simulink model "test_01_3d_veh_piby567_2018"  (R2018a)
settings: Solver=FixedStepAuto  StartTime=0.0  StopTime=50  FixedStep=0.1  RelTol=1e-3
values from neighbouring files (symbols this model uses):
  boundary = 0.1    [piby5tunnel.m]
  d_star = 0.6    [piby5tunnel.m]
  delta_arrow = 0.0295    [piby5tunnel.m]
  dtr = 7.3    [piby5tunnel.m]
  mu = 0.1    [piby5tunnel.m]
  N_n_p = zeros(slice,3)    [piby5tunnel.m]
  N_nfinal = zeros(slice-1,3*sides)    [piby5tunnel.m]
  P_c_final = zeros(slice-1,3*sides)    [piby5tunnel.m]
  sides = 8    [piby5tunnel.m]
  sigma = 0.005    [piby5tunnel.m]
  sum_ovf = zeros(slice,3)    [piby5tunnel.m]
  ubar = 1.5    [piby5tunnel.m]
  Ud = 1.485    [piby5tunnel.m]
  us = 1    [piby5tunnel.m]
  Vd = 1    [piby5tunnel.m]
  vehicle_velocity = 1    [piby5tunnel.m]
  x_0 = 30    [piby5tunnel.m]
  y_0 = 0    [piby5tunnel.m]
  z_0 = 0    [piby5tunnel.m]
libraries: vrlib x1, simulink x1
settings Model: Creator=satis  LastModifiedBy=Rasmus Visgaard

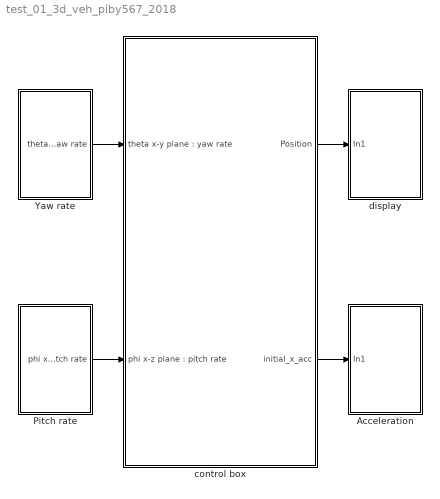
== system test_01_3d_veh_piby567_2018 ==
  "Acceleration " : Subsystem
  Pitch rate : Subsystem
  Yaw rate : Subsystem
  control box : Subsystem
  display : Subsystem
  wires:
  control box/1(Position) -> display/1(In1)
  Yaw rate/1("theta x-y plane : yaw rate") -> control box/1("theta x-y plane : yaw rate")
  Pitch rate/1("phi x-z plane : pitch rate") -> control box/2("phi x-z plane : pitch rate")
  control box/2(initial_x_acc) -> "Acceleration "/1(In1)

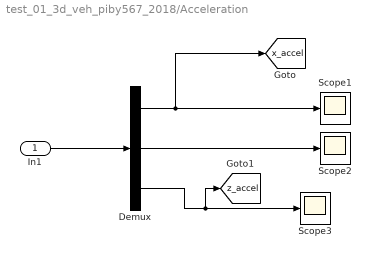
== system test_01_3d_veh_piby567_2018/Acceleration  ==
  In1 : Inport
  Demux : Demux  Outputs=3
  Scope1 : Scope
  Scope2 : Scope
  Scope3 : Scope
  tag scope: x_accel=global, z_accel=global
  wires:
  Demux/2 -> Scope2/1
  Demux/1 -> [x_accel], Scope1/1
  Demux/3 -> [z_accel], Scope3/1
  In1/1 -> Demux/1

== system test_01_3d_veh_piby567_2018/Pitch rate ==
  Constant4 : Constant  Value=0
  Step1 : Step  Time=0.1  SampleTime=0
  Switch1 : Switch  Criteria=u2 > Threshold
  "phi x-z plane : pitch rate" : Outport  VectorParamsAs1DForOutWhenUnconnected=off
  wires:
  Step1/1 -> Switch1/2
  Constant4/1 -> Switch1/3  "theta x-z plane : pitch rate"
  Switch1/1 -> "phi x-z plane : pitch rate"/1  "phi x-z plane : pitch rate"
  [z_accel] -> Switch1/1

== system test_01_3d_veh_piby567_2018/Yaw rate ==
  Constant2 : Constant  Value=0
  Step : Step  Time=0.1  SampleTime=0
  Switch : Switch  Criteria=u2 > Threshold
  "theta x-y plane : yaw rate" : Outport  VectorParamsAs1DForOutWhenUnconnected=off
  wires:
  Switch/1 -> "theta x-y plane : yaw rate"/1  "theta x-y plane : yaw rate"
  [x_accel] -> Switch/1
  Constant2/1 -> Switch/3  "theta x-y plane : yaw rate"
  Step/1 -> Switch/2

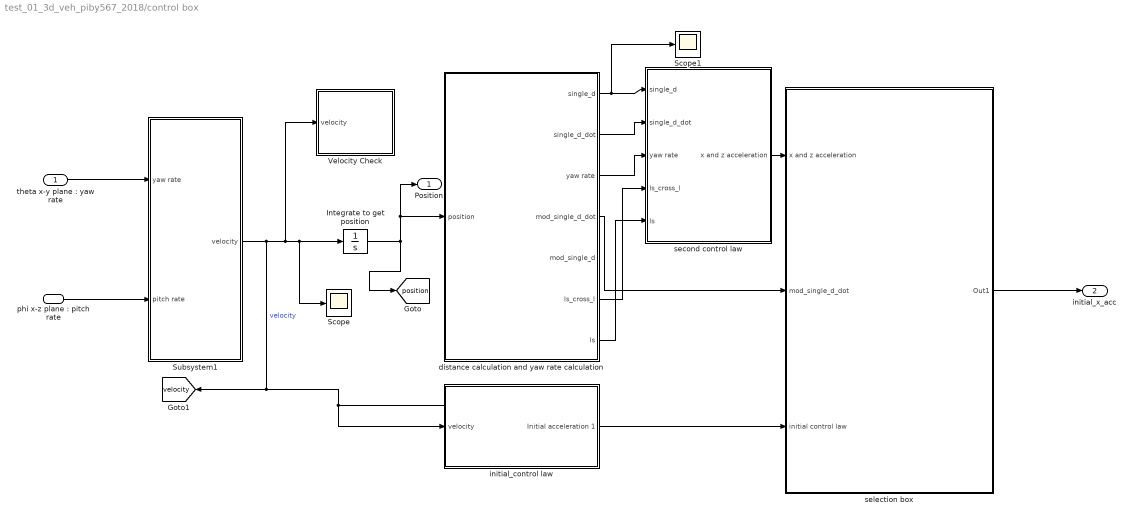
== system test_01_3d_veh_piby567_2018/control box ==
  "theta x-y plane : yaw rate" : Inport
  "phi x-z plane : pitch rate" : Inport  Port=2
  Integrate to get position : Integrator  InitialCondition=[x_0 z_0 y_0]
  Scope : Scope
  Scope1 : Scope
  Subsystem1 : Subsystem
  "Velocity Check " : Subsystem
  "distance calculation and yaw rate calculation " : Subsystem
  initial_control law : Subsystem
  second control law : Subsystem
  "selection box " : Subsystem
  Position : Outport  VectorParamsAs1DForOutWhenUnconnected=off
  initial_x_acc : Outport  Port=2  VectorParamsAs1DForOutWhenUnconnected=off
  tag scope: position=global, velocity=global
  wires:
  Subsystem1/1(velocity) -> initial_control law/1(velocity), [velocity], Scope/1, Integrate to get position/1, "Velocity Check "/1(velocity)  "velocity"
  "theta x-y plane : yaw rate"/1 -> Subsystem1/1("yaw rate ")
  "phi x-z plane : pitch rate"/1 -> Subsystem1/2(pitch rate)
  Integrate to get position/1 -> [position], Position/1, "distance calculation and yaw rate calculation "/1(position)
  "selection box "/1(Out1) -> initial_x_acc/1
  second control law/1(x and z acceleration) -> "selection box "/1(x and z acceleration)
  "distance calculation and yaw rate calculation "/1(single_d) -> Scope1/1, second control law/1(single_d)
  "distance calculation and yaw rate calculation "/2(single_d_dot) -> second control law/2(single_d_dot)
  "distance calculation and yaw rate calculation "/4(mod_single_d_dot) -> "selection box "/2(mod_single_d_dot)
  "distance calculation and yaw rate calculation "/3(yaw rate) -> second control law/3(yaw rate)
  "distance calculation and yaw rate calculation "/6(ls_cross_l) -> second control law/4(ls_cross_l)
  "distance calculation and yaw rate calculation "/7(ls) -> second control law/5(ls)
  initial_control law/1(Initial acceleration 1) -> "selection box "/3(initial control law)

== system test_01_3d_veh_piby567_2018/display ==
  In1 : Inport
  Demux : Demux  Outputs=3
  Scope10 : Scope
  Scope11 : Scope
  Scope12 : Scope
  wires:
  Demux/1 -> Scope10/1
  Demux/2 -> Scope11/1
  Demux/3 -> Scope12/1
  In1/1 -> Demux/1

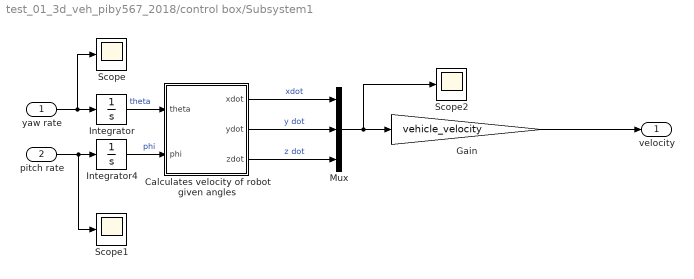
== system test_01_3d_veh_piby567_2018/control box/Subsystem1 ==
  "yaw rate " : Inport
  pitch rate : Inport  Port=2
  Calculates velocity of robot given angles : MATLAB Function  TreatAsAtomicUnit=on
  Gain : Gain  Gain=vehicle_velocity
  Integrator : Integrator
  Integrator4 : Integrator
  Mux : Mux  Inputs=3
  Scope : Scope
  Scope1 : Scope
  Scope2 : Scope
  velocity : Outport  VectorParamsAs1DForOutWhenUnconnected=off
  wires:
  Integrator4/1 -> Calculates velocity of robot given angles/2(phi)  "phi"
  Calculates velocity of robot given angles/1(xdot) -> Mux/1  "xdot"
  Integrator/1 -> Calculates velocity of robot given angles/1(theta)  "theta"
  Calculates velocity of robot given angles/2(ydot) -> Mux/2  "y dot"
  pitch rate/1 -> Scope1/1, Integrator4/1
  "yaw rate "/1 -> Scope/1, Integrator/1
  Calculates velocity of robot given angles/3(zdot) -> Mux/3  "z dot"
  Gain/1 -> velocity/1
  Mux/1 -> Scope2/1, Gain/1

== system test_01_3d_veh_piby567_2018/control box/Velocity Check  ==
  velocity : Inport
  Scope : Scope
  norm of velocity : Subsystem
  wires:
  norm of velocity/1(Out1) -> Scope/1
  velocity/1 -> norm of velocity/1(In1)

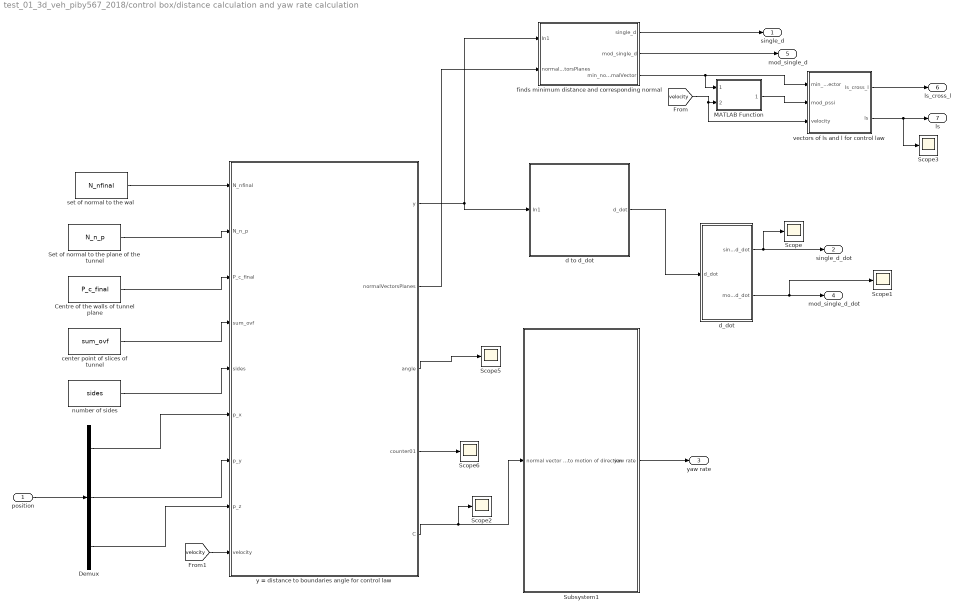
== system test_01_3d_veh_piby567_2018/control box/distance calculation and yaw rate calculation  ==
  position : Inport
  Centre of the walls of tunnel plane : Constant  Value=P_c_final  VectorParams1D=off
  Demux : Demux  Outputs=3
  MATLAB Function : MATLAB Function  TreatAsAtomicUnit=on
  Scope{,1..3,5..6} (6 alike) : Scope
  Set of normal to the plane of the tunnel : Constant  Value=N_n_p  VectorParams1D=off
  Subsystem1 : Subsystem
  center point of slices of tunnel : Constant  Value=sum_ovf  VectorParams1D=off
  d to d_dot : Subsystem
  d_dot : Subsystem
  finds minimum distance and corresponding normal : Subsystem
  number of sides : Constant  Value=sides
  set of normal to the wal : Constant  Value=N_nfinal  VectorParams1D=off
  vectors of ls and l for control law : MATLAB Function  TreatAsAtomicUnit=on
  "y = distance to boundaries angle for control law " : MATLAB Function  TreatAsAtomicUnit=on
  single_d : Outport  VectorParamsAs1DForOutWhenUnconnected=off
  single_d_dot : Outport  Port=2  VectorParamsAs1DForOutWhenUnconnected=off
  yaw rate : Outport  Port=3  VectorParamsAs1DForOutWhenUnconnected=off
  mod_single_d_dot : Outport  Port=4  VectorParamsAs1DForOutWhenUnconnected=off
  mod_single_d : Outport  Port=5  VectorParamsAs1DForOutWhenUnconnected=off
  ls_cross_l : Outport  Port=6
  ls : Outport  Port=7
  wires:
  set of normal to the wal/1 -> "y = distance to boundaries angle for control law "/1(N_nfinal)
  Centre of the walls of tunnel plane/1 -> "y = distance to boundaries angle for control law "/3(P_c_final)
  Set of normal to the plane of the tunnel/1 -> "y = distance to boundaries angle for control law "/2(N_n_p)
  center point of slices of tunnel/1 -> "y = distance to boundaries angle for control law "/4(sum_ovf)
  number of sides/1 -> "y = distance to boundaries angle for control law "/5(sides)
  position/1 -> Demux/1
  "y = distance to boundaries angle for control law "/1(y) -> d to d_dot/1(In1), finds minimum distance and corresponding normal/1(In1)
  Demux/1 -> "y = distance to boundaries angle for control law "/6(p_x)
  Demux/2 -> "y = distance to boundaries angle for control law "/7(p_y)
  Demux/3 -> "y = distance to boundaries angle for control law "/8(p_z)
  d to d_dot/1(d_dot) -> d_dot/1(d_dot)
  "y = distance to boundaries angle for control law "/3(angle) -> Scope5/1
  "y = distance to boundaries angle for control law "/4(counter01) -> Scope6/1
  "y = distance to boundaries angle for control law "/5(C) -> Scope2/1, Subsystem1/1(normal vector to motion of direction)
  Subsystem1/1(yaw rate) -> yaw rate/1
  finds minimum distance and corresponding normal/1(single_d) -> single_d/1
  finds minimum distance and corresponding normal/2(mod_single_d) -> mod_single_d/1
  d_dot/1(single_d_dot) -> Scope/1, single_d_dot/1
  d_dot/2(mod_single_d_dot) -> Scope1/1, mod_single_d_dot/1
  "y = distance to boundaries angle for control law "/2(normalVectorsPlanes) -> finds minimum distance and corresponding normal/2(normalVectorsPlanes)
  finds minimum distance and corresponding normal/3(min_normalVector) -> vectors of ls and l for control law/1(min_normalVector), MATLAB Function/1(min_normalVector)
  [velocity] -> MATLAB Function/2(velocity), vectors of ls and l for control law/3(velocity)
  MATLAB Function/1(mod_pssi) -> vectors of ls and l for control law/2(mod_pssi)
  vectors of ls and l for control law/1(ls_cross_l) -> ls_cross_l/1
  vectors of ls and l for control law/2(ls) -> Scope3/1, ls/1
  [velocity] -> "y = distance to boundaries angle for control law "/9(velocity)

== system test_01_3d_veh_piby567_2018/control box/initial_control law ==
  velocity : Inport
  Constant2 : Constant  Value=initial_normal_vector'
  Cross Product : vrlib/Utilities/Cross Product
      settings: SourceProductName=Simulink
  Gain : Gain  Gain=ubar
  Initial acceleration 1 : Outport  VectorParamsAs1DForOutWhenUnconnected=off
  wires:
  Cross Product/1 -> Gain/1
  velocity/1 -> Cross Product/1
  Constant2/1 -> Cross Product/2
  Gain/1 -> Initial acceleration 1/1

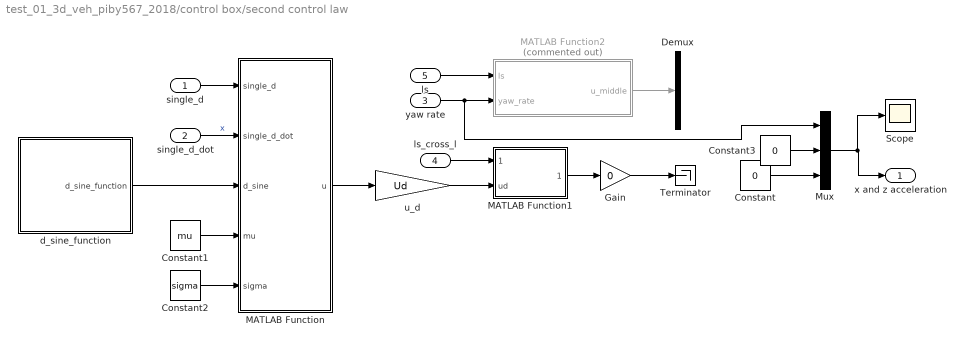
== system test_01_3d_veh_piby567_2018/control box/second control law ==
  single_d : Inport
  single_d_dot : Inport  Port=2
  yaw rate : Inport  Port=3
  ls_cross_l : Inport  Port=4
  ls : Inport  Port=5
  Constant : Constant  Value=0
  Constant1 : Constant  Value=mu
  Constant2 : Constant  Value=sigma
  Constant3 : Constant  Value=0
  Demux : Demux  Outputs=3
  Gain : Gain  Gain=0
  MATLAB Function : MATLAB Function  TreatAsAtomicUnit=on
  MATLAB Function1 : MATLAB Function  TreatAsAtomicUnit=on
  MATLAB Function2 : MATLAB Function  Commented=on  TreatAsAtomicUnit=on
  Mux : Mux  Inputs=3
  Scope : Scope
  Terminator : Terminator
  d_sine_function : Subsystem
  u_d : Gain  Gain=Ud
  x and z acceleration : Outport  VectorParamsAs1DForOutWhenUnconnected=off
  wires:
  single_d/1 -> MATLAB Function/1(single_d)
  Constant1/1 -> MATLAB Function/4(mu)
  Constant2/1 -> MATLAB Function/5(sigma)
  MATLAB Function/1(u) -> u_d/1
  d_sine_function/1(d_sine_function) -> MATLAB Function/3(d_sine)
  single_d_dot/1 -> MATLAB Function/2(single_d_dot)  "x"
  u_d/1 -> MATLAB Function1/2(ud)
  ls_cross_l/1 -> MATLAB Function1/1(ls_cross_l)
  ls/1 -> MATLAB Function2/1(ls)
  yaw rate/1 -> Mux/1, MATLAB Function2/2(yaw_rate)
  MATLAB Function2/1(u_middle) -> Demux/1
  MATLAB Function1/1(u_boundary) -> Gain/1
  Gain/1 -> Terminator/1
  Constant/1 -> Mux/3
  Constant3/1 -> Mux/2
  Mux/1 -> Scope/1, x and z acceleration/1

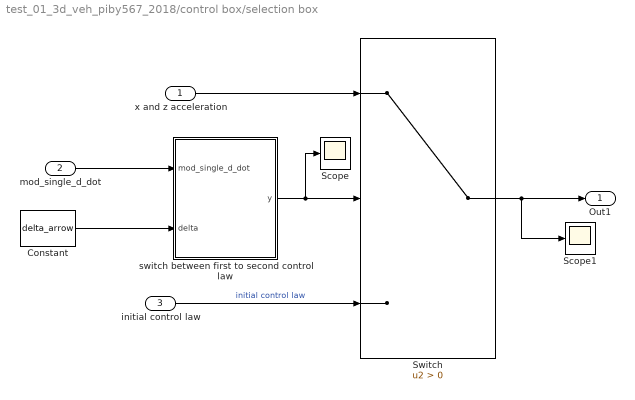
== system test_01_3d_veh_piby567_2018/control box/selection box  ==
  x and z acceleration : Inport
  mod_single_d_dot : Inport  Port=2
  initial control law : Inport  Port=3
  Constant : Constant  Value=delta_arrow
  Scope : Scope
  Scope1 : Scope
  Switch : Switch  Criteria=u2 > Threshold
  switch between first to second control law : MATLAB Function  TreatAsAtomicUnit=on
  Out1 : Outport  VectorParamsAs1DForOutWhenUnconnected=off
  wires:
  initial control law/1 -> Switch/3  "initial control law"
  x and z acceleration/1 -> Switch/1
  Constant/1 -> switch between first to second control law/2(delta)
  mod_single_d_dot/1 -> switch between first to second control law/1(mod_single_d_dot)
  Switch/1 -> Scope1/1, Out1/1
  switch between first to second control law/1(y) -> Scope/1, Switch/2

== system test_01_3d_veh_piby567_2018/control box/Velocity Check /norm of velocity ==
  In1 : Inport
  Takes the norm of input : MATLAB Function  TreatAsAtomicUnit=on
  Out1 : Outport  VectorParamsAs1DForOutWhenUnconnected=off
  wires:
  In1/1 -> Takes the norm of input/1(velocity)
  Takes the norm of input/1(normVelocity) -> Out1/1

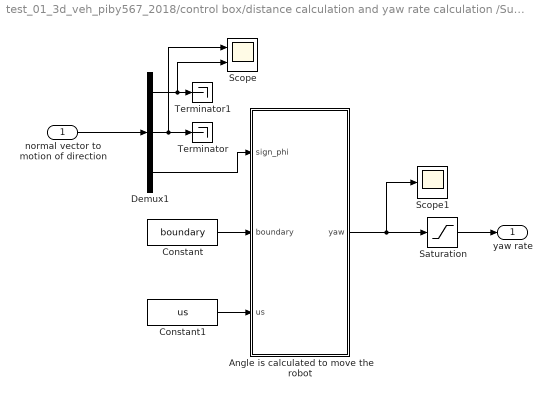
== system test_01_3d_veh_piby567_2018/control box/distance calculation and yaw rate calculation /Subsystem1 ==
  normal vector to motion of direction : Inport
  Angle is calculated to move the robot : MATLAB Function  TreatAsAtomicUnit=on
  Constant : Constant  Value=boundary
  Constant1 : Constant  Value=us
  Demux1 : Demux  Outputs=3
  Saturation : Saturate  UpperLimit=us  LowerLimit=-us
  Scope : Scope  NumInputPorts=2
  Scope1 : Scope
  Terminator : Terminator
  Terminator1 : Terminator
  yaw rate : Outport  VectorParamsAs1DForOutWhenUnconnected=off
  wires:
  Demux1/3 -> Angle is calculated to move the robot/1(sign_phi)
  normal vector to motion of direction/1 -> Demux1/1
  Angle is calculated to move the robot/1(yaw) -> Scope1/1, Saturation/1
  Demux1/2 -> Scope/1, Terminator/1
  Demux1/1 -> Scope/2, Terminator1/1
  Constant/1 -> Angle is calculated to move the robot/2(boundary)
  Saturation/1 -> yaw rate/1
  Constant1/1 -> Angle is calculated to move the robot/3(us)

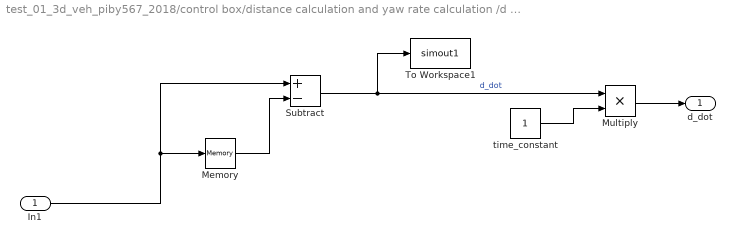
== system test_01_3d_veh_piby567_2018/control box/distance calculation and yaw rate calculation /d to d_dot ==
  In1 : Inport
  Memory : Memory
  Multiply : Product
  Subtract : Sum  Inputs=+-
  To Workspace1 : ToWorkspace  VariableName=simout1  SaveFormat=Timeseries  SampleTime=-1
  time_constant : Constant
  d_dot : Outport  VectorParamsAs1DForOutWhenUnconnected=off
  wires:
  Memory/1 -> Subtract/2
  In1/1 -> Subtract/1, Memory/1
  Subtract/1 -> To Workspace1/1, Multiply/1  "d_dot"
  time_constant/1 -> Multiply/2
  Multiply/1 -> d_dot/1

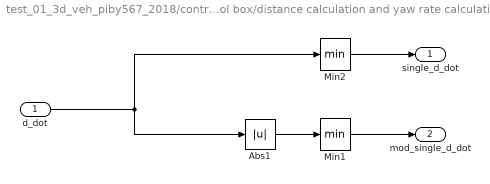
== system test_01_3d_veh_piby567_2018/control box/distance calculation and yaw rate calculation /d_dot ==
  d_dot : Inport
  Abs1 : Abs
  Min1 : MinMax
  Min2 : MinMax
  single_d_dot : Outport  VectorParamsAs1DForOutWhenUnconnected=off
  mod_single_d_dot : Outport  Port=2  VectorParamsAs1DForOutWhenUnconnected=off
  wires:
  Abs1/1 -> Min1/1
  Min1/1 -> mod_single_d_dot/1
  d_dot/1 -> Min2/1, Abs1/1
  Min2/1 -> single_d_dot/1

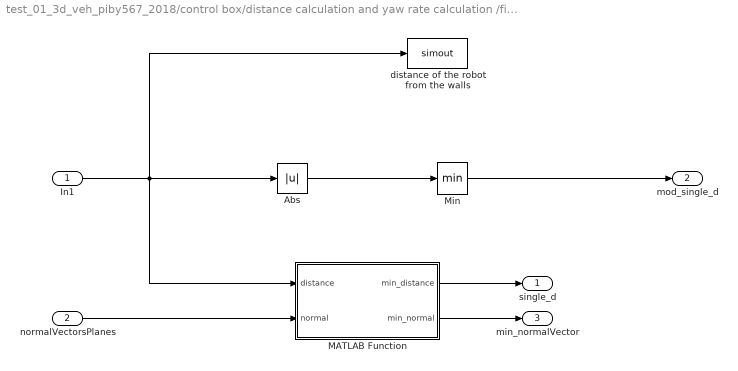
== system test_01_3d_veh_piby567_2018/control box/distance calculation and yaw rate calculation /finds minimum distance and corresponding normal ==
  In1 : Inport
  normalVectorsPlanes : Inport  Port=2
  Abs : Abs
  MATLAB Function : MATLAB Function  TreatAsAtomicUnit=on
  Min : MinMax
  distance of the robot from the walls : ToWorkspace  VariableName=simout  SaveFormat=Timeseries  SampleTime=-1
  single_d : Outport  VectorParamsAs1DForOutWhenUnconnected=off
  mod_single_d : Outport  Port=2  VectorParamsAs1DForOutWhenUnconnected=off
  min_normalVector : Outport  Port=3  VectorParamsAs1DForOutWhenUnconnected=off
  wires:
  Abs/1 -> Min/1
  In1/1 -> MATLAB Function/1(distance), distance of the robot from the walls/1, Abs/1
  Min/1 -> mod_single_d/1
  normalVectorsPlanes/1 -> MATLAB Function/2(normal)
  MATLAB Function/2(min_normal) -> min_normalVector/1
  MATLAB Function/1(min_distance) -> single_d/1

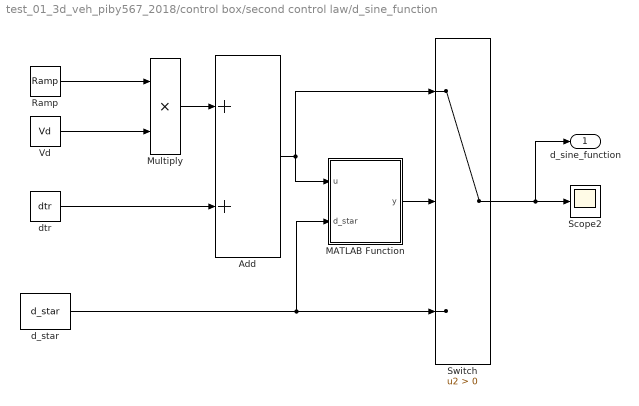
== system test_01_3d_veh_piby567_2018/control box/second control law/d_sine_function ==
  Add : Sum
  MATLAB Function : MATLAB Function  TreatAsAtomicUnit=on
  Multiply : Product
  Ramp : simulink/Sources/Ramp  slope=-1  start=0  InitialOutput=0
  Scope2 : Scope
  Switch : Switch  Criteria=u2 > Threshold
  Vd : Constant  Value=Vd
  d_star : Constant  Value=d_star
  dtr : Constant  Value=dtr
  d_sine_function : Outport  VectorParamsAs1DForOutWhenUnconnected=off
  wires:
  Multiply/1 -> Add/1
  d_star/1 -> MATLAB Function/2(d_star), Switch/3
  MATLAB Function/1(y) -> Switch/2
  Vd/1 -> Multiply/2
  Switch/1 -> d_sine_function/1, Scope2/1
  Add/1 -> MATLAB Function/1(u), Switch/1
  Ramp/1 -> Multiply/1
  dtr/1 -> Add/2

== matlab function test_01_3d_veh_piby567_2018/control box/second control law/d_sine_function/MATLAB Function ==
  data: u input; y output; d_star input
function y = fcn(u,d_star)
if u>d_star
   y=1; 
else
  y=0;
end

== matlab function test_01_3d_veh_piby567_2018/control box/distance calculation and yaw rate calculation /y = distance to boundaries angle for control law  ==
  data: N_nfinal input; N_n_p input; P_c_final input; y output; normalVectorsPlanes output; sum_ovf input; sides input; p_x input; p_y input; p_z input; angle output; counter01 output; C output; velocity input
function [y,normalVectorsPlanes,angle,counter01,C] = fcn(N_nfinal,N_n_p,P_c_final,sum_ovf,sides,p_x,p_y,p_z, velocity)
%distance from the sections
position=[p_x,p_y,p_z];
dis_arrs02=zeros(length(N_n_p),1);
%angle_arrs02=zeros(length(N_n_p),1);
%this loop calculates distance to 
for kk22=1:length(N_n_p)% as the robot will move forward the distance with the vertical plane will be positive
    a1=position-sum_ovf(kk22,:);
    b1=N_n_p(kk22,:);
    dis22=dot(a1,b1);
    %angle = atan2(norm(cross(a,b)), dot(a,b));
    dis_arrs02(kk22,1) =dis22;
    %angle_arrs02(kk22,1) =angle;
end
counter01=0;
for count=1:length(dis_arrs02)
    if(dis_arrs02(count,1)>=0)
        counter01=counter01+1;
    end
end
if counter01>=length(dis_arrs02)
    counter01=length(dis_arrs02)-1;
end

slice_num=counter01;
% a=position-sum_ovf(counter01,:);
%b=N_n_p(counter01,:);
b = sum_ovf(counter01+1,:)-sum_ovf(counter01,:);
C = cross(velocity,b);
angle = atan2(norm(cross(velocity,b)), dot(velocity,b)); %angle from (distance between center point of slice and vehicle) 
%to normal plane of slice

% C = cross(a,b);
% angle = atan2(norm(cross(a,b)), dot(a,b));

bound_dis1=zeros(8,1);
normal_distance = zeros(8,3);
for nn=1:sides
    normal_tmp=N_nfinal(slice_num,3*(nn-1)+1: 3*nn);
    point_tmp=P_c_final(slice_num,3*(nn-1)+1: 3*nn);
    dis3=dot(position-point_tmp,normal_tmp);
    bound_dis1(nn,1)=dis3;
    normal_distance(nn,1:3) = normal_tmp;
 end
%end
y=bound_dis1;
normalVectorsPlanes=normal_distance;

%plot3(position(1,1),position(1,2),position(1,3))

== matlab function test_01_3d_veh_piby567_2018/control box/selection box /switch between first to second control law ==
  settings: updateMethod=DISCRETE  sampleTime=0.1
  data: mod_single_d_dot input; y output; delta input
function y = fcn(mod_single_d_dot,delta)
persistent n;
if isempty(n)
    n=1;
end

switch n
    case 1
        if mod_single_d_dot<delta
            y=1;
            n=2;
        else
            y=0;
        end
    case 2
        y=1;
    otherwise
        y=0;
end
end

== matlab function test_01_3d_veh_piby567_2018/control box/Subsystem1/Calculates velocity of robot given angles ==
  data: theta input; xdot output; phi input; ydot output; zdot output
function [xdot, ydot, zdot] = fcn(theta, phi)

xdot = sin(theta)*cos(phi); 
ydot = cos(theta)*cos(phi);
zdot = sin(phi);

== matlab function test_01_3d_veh_piby567_2018/control box/second control law/MATLAB Function ==
  data: single_d input; u output; single_d_dot input; d_sine input; mu input; sigma input
function u = fcn(single_d,single_d_dot,d_sine, mu, sigma)

a = (single_d-d_sine)/sigma;

if a >= mu
a = mu;
elseif a  <= -mu
a = -mu;
else
end

u = sign(single_d_dot+a);

== matlab function test_01_3d_veh_piby567_2018/control box/distance calculation and yaw rate calculation /Subsystem1/Angle is calculated to move the robot ==
  data: yaw output; sign_phi input; boundary input; us input
function yaw = fcn(sign_phi,boundary,us)
if sign_phi > 0
    yaw=-us;
elseif sign_phi < 0
    yaw=us;   
else 
    yaw = 0;
end

%yaw = -sign_phi/boundary;

== matlab function test_01_3d_veh_piby567_2018/control box/Velocity Check /norm of velocity/Takes the norm of input ==
  data: velocity input; normVelocity output
function normVelocity = fcn(velocity)

normVelocity = norm(velocity);

== matlab function test_01_3d_veh_piby567_2018/control box/distance calculation and yaw rate calculation /finds minimum distance and corresponding normal/MATLAB Function ==
  data: distance input; min_distance output; normal input; min_normal output
function [min_distance,min_normal] = fcn(distance,normal)

[min_distance,index] = min(distance);
min_normal = normal(index,1:3);

== matlab function test_01_3d_veh_piby567_2018/control box/distance calculation and yaw rate calculation /MATLAB Function ==
  data: min_normalVector input; mod_pssi output; velocity input
function mod_pssi = fcn(min_normalVector,velocity)
%angle = atan2(norm(cross(a,b)), dot(a,b));

%normalize normal vector
norm_min_normalVector = min_normalVector/norm(min_normalVector);

%angle between velocity direction and normal to plane (side)
pssi = atan2(norm(cross(norm_min_normalVector',velocity)),dot(norm_min_normalVector',velocity));
mod_pssi = abs(sin(pssi)); %mod of sin(angle)

== matlab function test_01_3d_veh_piby567_2018/control box/distance calculation and yaw rate calculation /vectors of ls and l for control law ==
  data: min_normalVector input; mod_pssi input; ls_cross_l output; velocity input; ls output
function [ls_cross_l, ls] = fcn(min_normalVector, mod_pssi, velocity)

norm_min_normalVector = min_normalVector/norm(min_normalVector);

ls = cross(velocity,norm_min_normalVector)/mod_pssi;

ls_cross_l = cross(cross(velocity,norm_min_normalVector),velocity)/mod_pssi;

== matlab function test_01_3d_veh_piby567_2018/control box/second control law/MATLAB Function1 ==
  data: ls_cross_l input; ud input; u_boundary output
function u_boundary = fcn(ls_cross_l,ud)

u_boundary = ud*ls_cross_l;

== matlab function test_01_3d_veh_piby567_2018/control box/second control law/MATLAB Function2 ==
  data: ls input; u_middle output; yaw_rate input
function u_middle = fcn(ls,yaw_rate)

%u_middle = yaw_rate*ls;
u_middle = yaw_rate;
